simulink model "demoDisplay"  (R2018b)
settings: Solver=FixedStepAuto  StartTime=0.0  StopTime=20  FixedStep=.01  RelTol=1e-3
undefined symbols (not defined in the file): CR, LF, serial
libraries: instrumentlib x2
settings Model: EnablePacing=on  Creator=nickanselmo  LastModifiedBy=nickanselmo

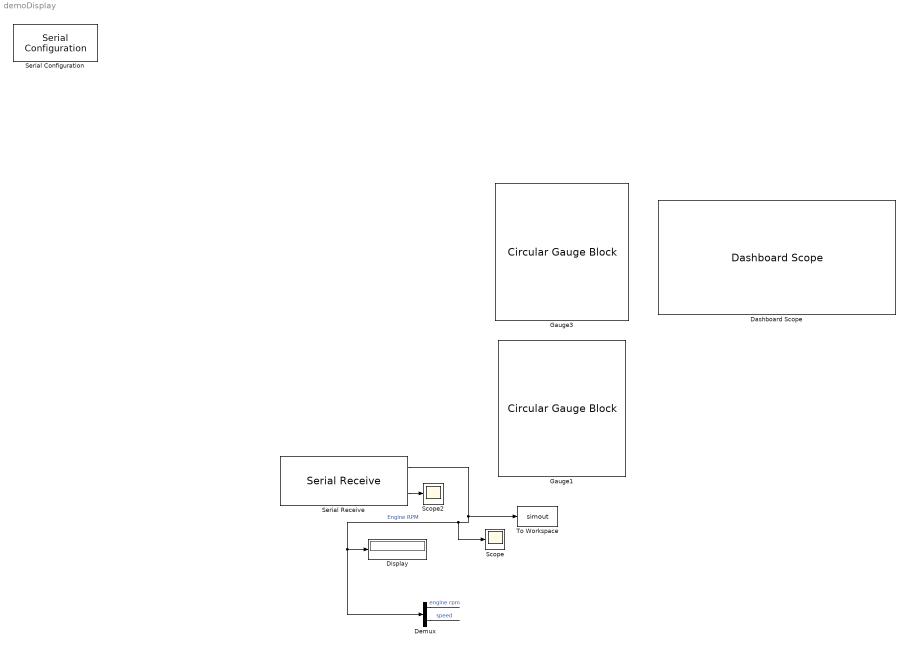
== system demoDisplay ==
  Dashboard Scope : DashboardScope  WebBlockId=11  Ymin=0  Ymax=3800
  Demux : Demux  Outputs=2
  Display : Display
  Gauge1 : CircularGaugeBlock  WebBlockId=20  ScaleMax=4000
  Gauge3 : CircularGaugeBlock  WebBlockId=25  ScaleMax=4000
  Scope : Scope
  Scope2 : Scope
  Serial Configuration : instrumentlib/Serial Configuration  Priority=-200000  ComPortMenu=/dev/cu.usbmodem14101  ComPort=/dev/cu.usbmodem14101  ObjConstructor=serial('/dev/cu.usbmodem14101');  BaudRate=115200  DataBits=8  Parity=none  StopBits=1  FlowControl=none  Timeout=10  ByteOrder=BigEndian
  Serial Receive : instrumentlib/Serial Receive  ComPortMenu=/dev/cu.usbmodem14101  ComPort=/dev/cu.usbmodem14101  ObjConstructor=serial('/dev/cu.usbmodem14101');  Header=()  Terminator=CR/LF ('\r\n')  DataSize=2  DataType=int16  EnableBlockingMode=off  ActionDataUnavailable=Output last received value  CustomValue=0  SampleTime=.01
  To Workspace : ToWorkspace  VariableName=simout  SaveFormat=Timeseries  SampleTime=-1
  wires:
  Serial Receive/1 -> To Workspace/1, Scope/1, Demux/1, Display/1  "Engine RPM"
  Demux/1 -> ?  "engine rpm"
  Demux/2 -> ?  "speed"
  Serial Receive/2 -> Scope2/1
